simulink model "simulink_afbs_test"  (R2015a)
settings: Solver=ode45  StartTime=0.0  StopTime=1  FixedStep=0.1  RelTol=1e-4
settings Model: Creator=Xiaotian  LastModifiedBy=Xiaotian

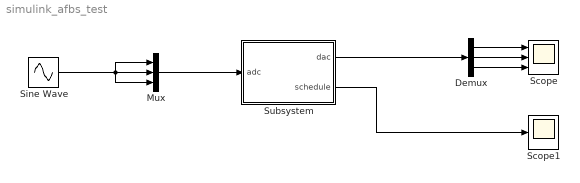
== system simulink_afbs_test ==
  Demux : Demux  Outputs=3
  Mux : Mux  Inputs=3
  Scope : Scope  NumInputPorts=3
      settings: YMin=-5~-5~-5  YMax=5~5~5
  Scope1 : Scope
  Sine Wave : Sin  Frequency=2*3.14*1  SampleTime=0
  Subsystem : Subsystem  mask{Parameter2=on, Parameter3=0}
  wires:
  Sine Wave/1 -> Mux/3, Mux/2, Mux/1
  Subsystem/1(dac) -> Demux/1
  Mux/1 -> Subsystem/1(adc)
  Demux/1 -> Scope/1
  Demux/2 -> Scope/2
  Demux/3 -> Scope/3
  Subsystem/2(schedule) -> Scope1/1

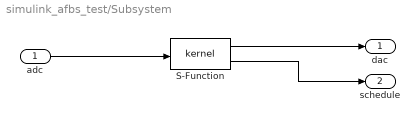
== system simulink_afbs_test/Subsystem ==
  adc : Inport
  S-Function : S-Function  FunctionName=kernel
  dac : Outport
  schedule : Outport  Port=2
  wires:
  adc/1 -> S-Function/1
  S-Function/1 -> dac/1
  S-Function/2 -> schedule/1
